simulink model "etc_throttle_start"  (R2018a)
settings: Solver=ode45  StartTime=0.0  StopTime=20.0  RelTol=1e-3  EnableMultiTasking=on
PreLoadFcn:
  | etc_plant_data;
values from neighbouring files (symbols this model uses):
  degConv = 180/pi    (= 57.2957795131)    [etc_all_data.m]
undefined symbols (not defined in the file or in its folder): Cs, J, Kd, Ks, theta_eq
Description:
  | This is my help
settings Model: ParamWorkspaceSource=ReferencedWorkspace  Creator=koliver  LastModifiedBy=bneiswan
settings DataIOCC: ExternalInput=[t, direction, duty]  LimitDataPoints=on  LoadExternalInput=on  SaveFormat=Array  SignalLoggingName=sigsOut
settings OptimizationCC: DefaultParameterBehavior=Inlined  ExpressionDepthLimit=2147483647  InitFltsAndDblsToZero=on  LifeSpan=inf
settings DebuggingCC: SaveWithParameterizedLinksMsg=none  UnderspecifiedInitializationDetection=Classic  MergeDetectMultiDrivingBlocksExec=none  MultiTaskDSMMsg=warning  MultiTaskCondExecSysMsg=none  ParameterPrecisionLossMsg=none  FcnCallInpInsideContextMsg=warning  AllowSymbolicDim=off  StateNameClashWarn=warning  SFUnexpectedBacktrackingDiag=warning  SFNoUnconditionalDefaultTransitionDiag=warning  SFExecutionAtInitializationDiag=none
settings HardwareCC: ProdBitPerPointer=32  ProdBitPerSizeT=32  ProdBitPerPtrDiffT=32  ProdLargestAtomicFloat=None  ProdIntDivRoundTo=Undefined  ProdEndianess=Unspecified  ProdWordSize=32  ProdHWDeviceType=32-bit Generic  TargetIntDivRoundTo=Zero  TargetEndianess=BigEndian  TargetHWDeviceType=Motorola PowerPC
settings ModelReferenceCC: ModelReferenceNumInstancesAllowed=Single  PropagateSignalLabelsOutOfModel=off
settings SFSimCC: SimParseCustomCode=off
settings CodeAppCC: StateflowObjectComments=on
settings GRTTargetCC: TargetFcnLib=ansi_tfl_tmw.mat  TargetLangStandard=C89/C90 (ANSI)  GeneratePreprocessorConditionals=Disable all  CombineOutputUpdateFcns=off  GRTInterface=on
settings ConfigComp: CovMetricSettings=dw  CovHtmlReporting=on  CovSaveCumulativeToWorkspaceVar=on  CovSaveSingleToWorkspaceVar=on  CovExternalEMLEnable=off  CovSFcnEnable=off

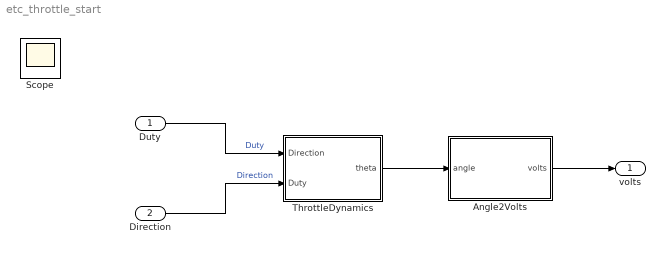
== system etc_throttle_start ==
  Duty : Inport
  Direction : Inport  Port=2
  Angle2Volts : Subsystem
  ThrottleDynamics : Subsystem
  volts : Outport
  Scope : Scope
  wires:
  ThrottleDynamics/1(theta) -> Angle2Volts/1("angle ")
  Angle2Volts/1(volts) -> volts/1
  Duty/1 -> ThrottleDynamics/1(Direction)  "Duty"
  Direction/1 -> ThrottleDynamics/2(Duty)  "Direction"

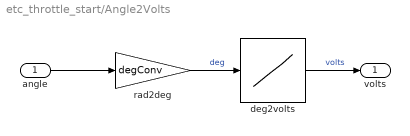
== system etc_throttle_start/Angle2Volts ==
  "angle " : Inport
  deg2volts : Lookup_n-D  NumberOfTableDimensions=1  BreakpointsForDimension1=[0 90]  Table=[0.5 4.5]  RndMeth=Simplest  InputSameDT=on
  rad2deg : Gain  Gain=degConv  SaturateOnIntegerOverflow=on  OutDataTypeStr=Inherit: Same as input  ParamDataTypeStr=Inherit: Same as input
  volts : Outport
  wires:
  rad2deg/1 -> deg2volts/1  "deg"
  deg2volts/1 -> volts/1  "volts"
  "angle "/1 -> rad2deg/1

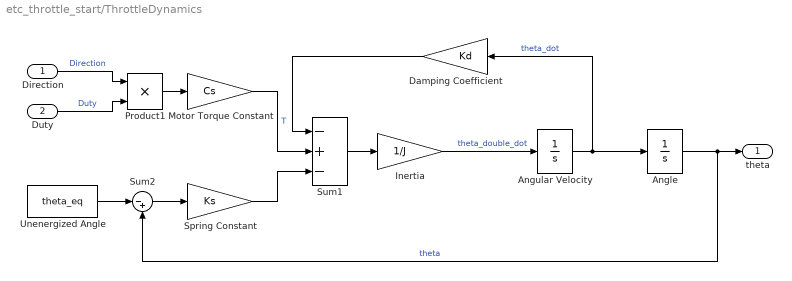
== system etc_throttle_start/ThrottleDynamics ==
  Direction : Inport
  Duty : Inport  Port=2
  Angle : Integrator  InitialCondition=pi/6  LimitOutput=on  UpperSaturationLimit=pi/2  LowerSaturationLimit=0
      settings: AttributesFormatString=Initial condition: %<InitialCondition>\n%<LowerSaturationLimit> <= theta <= %<UpperSaturationLimit>
  Angular Velocity : Integrator
      settings: AttributesFormatString=Initial condition: %<InitialCondition>
  Damping Coefficient : Gain  Gain=Kd  SaturateOnIntegerOverflow=on  OutDataTypeStr=Inherit: Same as input  ParamDataTypeStr=Inherit: Same as input
  Inertia : Gain  Gain=1/J  SaturateOnIntegerOverflow=on  OutDataTypeStr=Inherit: Same as input  ParamDataTypeStr=Inherit: Same as input
  Motor Torque Constant : Gain  Gain=Cs  SaturateOnIntegerOverflow=on  OutDataTypeStr=Inherit: Same as input  ParamDataTypeStr=Inherit: Same as input
  Product1 : Product  SaturateOnIntegerOverflow=on  OutDataTypeStr=Inherit: Same as first input
  Spring Constant : Gain  Gain=Ks  SaturateOnIntegerOverflow=on  OutDataTypeStr=Inherit: Same as input  ParamDataTypeStr=Inherit: Same as input
  Sum1 : Sum  Inputs=-+-  SaturateOnIntegerOverflow=on
  Sum2 : Sum  Inputs=|-+  SaturateOnIntegerOverflow=on
  Unenergized Angle : Constant  Value=theta_eq
  theta : Outport
  wires:
  Product1/1 -> Motor Torque Constant/1
  Unenergized Angle/1 -> Sum2/1
  Sum2/1 -> Spring Constant/1
  Angle/1 -> theta/1, Sum2/2  "theta"
  Angular Velocity/1 -> Angle/1, Damping Coefficient/1  "theta_dot"
  Inertia/1 -> Angular Velocity/1  "theta_double_dot"
  Sum1/1 -> Inertia/1
  Direction/1 -> Product1/1  "Direction"
  Duty/1 -> Product1/2  "Duty"
  Motor Torque Constant/1 -> Sum1/2  "T"
  Damping Coefficient/1 -> Sum1/1
  Spring Constant/1 -> Sum1/3
